simulink library "ESSLibrary"  (R2020a)
settings: Solver=VariableStepAuto  StartTime=0.0  StopTime=10.0  RelTol=1e-3
libraries: $bdroot x82, powerlib_meascontrol x10, simulink x7
(part 3 of 7)

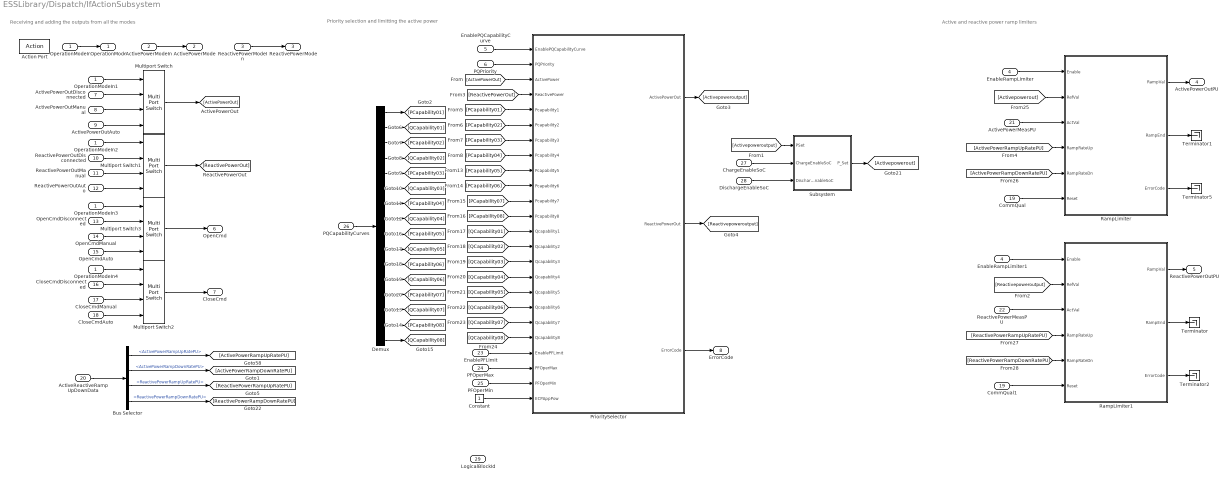
== system ESSLibrary/Dispatch/IfActionSubsystem ==
  note: Active and reactive power ramp limiters
  note: Priority selection and limitting the active power
  note: Receiving and adding the outputs from all the modes
  OperationModeIn : Inport  OutDataTypeStr=int8
  ActivePowerModeIn : Inport  Port=2
  ReactivePowerModeIn : Inport  Port=3
  EnableRampLimiter : Inport  Port=4
  EnablePQCapabilityCurve : Inport  Port=5
  PQPriority : Inport  Port=6
  ActivePowerOutDisconnected : Inport  Port=7
  ActivePowerOutManual : Inport  Port=8
  ActivePowerOutAuto : Inport  Port=9
  ReactivePowerOutDisconnected : Inport  Port=10
  ReactivePowerOutManual : Inport  Port=11
  ReactivePowerOutAuto : Inport  Port=12
  OpenCmdDisconnected : Inport  Port=13
  OpenCmdManual : Inport  Port=14
  OpenCmdAuto : Inport  Port=15
  CloseCmdDisconnected : Inport  Port=16
  CloseCmdManual : Inport  Port=17
  CloseCmdAuto : Inport  Port=18
  CommQual : Inport  Port=19
  ActiveReactiveRampUpDownData : Inport  Port=20  OutDataTypeStr=Bus: ActiveReactiveRampUpDownData
  ActivePowerMeasPU : Inport  Port=21
  ReactivePowerMeasPU : Inport  Port=22
  EnablePFLimit : Inport  Port=23
  PFOperMax : Inport  Port=24
  PFOperMin : Inport  Port=25
  PQCapabilityCurves : Inport  Port=26  OutDataTypeStr=double
  ChargeEnableSoC : Inport  Port=27
  DischargeEnableSoC : Inport  Port=28
  LogicalBlockId : Inport  Port=29
  Action Port : ActionPort
  Bus Selector : BusSelector  OutputSignals=ActivePowerRampUpRatePU,ActivePowerRampDownRatePU,ReactivePowerRampUpRatePU,ReactivePowerRampDownRatePU
  CommQual1 : InportShadow  Port=19
  Constant : Constant  OutDataTypeStr=double  SampleTime=-1
  Demux : Demux  Outputs=16
  EnableRampLimiter1 : InportShadow  Port=4
  Multiport Switch{,1..3} (4 alike) : MultiPortSwitch
  OperationModeIn{1..4} (4 alike) : InportShadow  OutDataTypeStr=int8
  PrioritySelector : Subsystem
  RampLimiter : MATLAB Function  TreatAsAtomicUnit=on
  RampLimiter1 : MATLAB Function  TreatAsAtomicUnit=on
  Subsystem : Subsystem
  Terminator{,1..2,5} (4 alike) : Terminator
  OperationMode : Outport
  ActivePowerMode : Outport  Port=2
  ReactivePowerMode : Outport  Port=3
  ActivePowerOutPU : Outport  Port=4
  ReactivePowerOutPU : Outport  Port=5
  OpenCmd : Outport  Port=6
  CloseCmd : Outport  Port=7
  ErrorCode : Outport  Port=8
  wires:
  Multiport Switch/1 -> [ActivePowerOut]
  Multiport Switch3/1 -> OpenCmd/1
  Multiport Switch1/1 -> [ReactivePowerOut]
  Multiport Switch2/1 -> CloseCmd/1
  OperationModeIn/1 -> OperationMode/1
  ActivePowerOutDisconnected/1 -> Multiport Switch/2
  ActivePowerOutManual/1 -> Multiport Switch/3
  ActivePowerOutAuto/1 -> Multiport Switch/4
  ReactivePowerOutAuto/1 -> Multiport Switch1/4
  ReactivePowerOutManual/1 -> Multiport Switch1/3
  ReactivePowerOutDisconnected/1 -> Multiport Switch1/2
  OpenCmdDisconnected/1 -> Multiport Switch3/2
  OpenCmdManual/1 -> Multiport Switch3/3
  OpenCmdAuto/1 -> Multiport Switch3/4
  CloseCmdAuto/1 -> Multiport Switch2/4
  CloseCmdManual/1 -> Multiport Switch2/3
  CloseCmdDisconnected/1 -> Multiport Switch2/2
  EnablePQCapabilityCurve/1 -> PrioritySelector/1(EnablePQCapabilityCurve)
  PQPriority/1 -> PrioritySelector/2(PQPriority)
  RampLimiter1/2(RampEnd) -> Terminator/1
  RampLimiter/3(ErrorCode) -> Terminator5/1
  RampLimiter/1(RampVal) -> ActivePowerOutPU/1
  EnableRampLimiter1/1 -> RampLimiter1/1(Enable)
  RampLimiter1/1(RampVal) -> ReactivePowerOutPU/1
  EnableRampLimiter/1 -> RampLimiter/1(Enable)
  PrioritySelector/1(ActivePowerOut) -> [Activepoweroutput]
  PrioritySelector/2(ReactivePowerOut) -> [Reactivepoweroutput]
  CommQual/1 -> RampLimiter/6(Reset)
  CommQual1/1 -> RampLimiter1/6(Reset)
  ActivePowerMeasPU/1 -> RampLimiter/3(ActVal)
  ReactivePowerMeasPU/1 -> RampLimiter1/3(ActVal)
  [ActivePowerOut] -> PrioritySelector/3(ActivePower)
  [ReactivePowerOut] -> PrioritySelector/4(ReactivePower)
  [ActivePowerRampUpRatePU] -> RampLimiter/4(RampRateUp)
  [ActivePowerRampDownRatePU] -> RampLimiter/5(RampRateDn)
  [ReactivePowerRampDownRatePU] -> RampLimiter1/5(RampRateDn)
  [ReactivePowerRampUpRatePU] -> RampLimiter1/4(RampRateUp)
  RampLimiter/2(RampEnd) -> Terminator1/1
  RampLimiter1/3(ErrorCode) -> Terminator2/1
  [Reactivepoweroutput] -> RampLimiter1/2(RefVal)
  EnablePFLimit/1 -> PrioritySelector/21(EnablePFLimit)
  PFOperMax/1 -> PrioritySelector/22(PFOperMax)
  PFOperMin/1 -> PrioritySelector/23(PFOperMin)
  PQCapabilityCurves/1 -> Demux/1
  Demux/1 -> [PCapability01]
  Demux/2 -> [QCapability01]
  Demux/3 -> [PCapability02]
  Demux/4 -> [QCapability02]
  Demux/5 -> [PCapability03]
  Demux/6 -> [QCapability03]
  Demux/7 -> [PCapability04]
  Demux/8 -> [QCapability04]
  Demux/9 -> [PCapability05]
  Demux/10 -> [QCapability05]
  Demux/11 -> [PCapability06]
  Demux/12 -> [QCapability06]
  Demux/13 -> [PCapability07]
  Demux/14 -> [QCapability07]
  Demux/15 -> [PCapability08]
  Demux/16 -> [QCapability08]
  [PCapability01] -> PrioritySelector/5(Pcapability1)
  [PCapability02] -> PrioritySelector/6(Pcapability2)
  [PCapability03] -> PrioritySelector/7(Pcapability3)
  [PCapability04] -> PrioritySelector/8(Pcapability4)
  [PCapability05] -> PrioritySelector/9(Pcapability5)
  [PCapability06] -> PrioritySelector/10(Pcapability6)
  [PCapability07] -> PrioritySelector/11(Pcapability7)
  [PCapability08] -> PrioritySelector/12(Pcapability8)
  [QCapability01] -> PrioritySelector/13(Qcapability1)
  [QCapability02] -> PrioritySelector/14(Qcapability2)
  [QCapability03] -> PrioritySelector/15(Qcapability3)
  [QCapability05] -> PrioritySelector/17(Qcapability5)
  [QCapability04] -> PrioritySelector/16(Qcapability4)
  [QCapability06] -> PrioritySelector/18(Qcapability6)
  [QCapability07] -> PrioritySelector/19(Qcapability7)
  [QCapability08] -> PrioritySelector/20(Qcapability8)
  [Activepoweroutput] -> Subsystem/1(PSet)
  ChargeEnableSoC/1 -> Subsystem/2(ChargeEnableSoC)
  DischargeEnableSoC/1 -> Subsystem/3(DischargeEnableSoC)
  [Activepowerout] -> RampLimiter/2(RefVal)
  PrioritySelector/3(ErrorCode) -> ErrorCode/1
  Subsystem/1(P_Set) -> [Activepowerout]
  ActivePowerModeIn/1 -> ActivePowerMode/1
  ReactivePowerModeIn/1 -> ReactivePowerMode/1
  Constant/1 -> PrioritySelector/24(ECPAppPow)
  OperationModeIn1/1 -> Multiport Switch/1
  OperationModeIn2/1 -> Multiport Switch1/1
  OperationModeIn3/1 -> Multiport Switch3/1
  OperationModeIn4/1 -> Multiport Switch2/1
  ActiveReactiveRampUpDownData/1 -> Bus Selector/1
  Bus Selector/1 -> [ActivePowerRampUpRatePU]  "<ActivePowerRampUpRatePU>"
  Bus Selector/2 -> [ActivePowerRampDownRatePU]  "<ActivePowerRampDownRatePU>"
  Bus Selector/3 -> [ReactivePowerRampUpRatePU]  "<ReactivePowerRampUpRatePU>"
  Bus Selector/4 -> [ReactivePowerRampDownRatePU]  "<ReactivePowerRampDownRatePU>"

== system ESSLibrary/Divider/ElseActionSubsystem ==
  Action Port : ActionPort
  Constant1 : Constant  Value=0  OutDataTypeStr=int64  SampleTime=-1
  Constant11 : Constant  Value=0  OutDataTypeStr=boolean  SampleTime=-1
  Constant2 : Constant  Value=0  OutDataTypeStr=double  SampleTime=-1
  Quality : Outport  OutDataTypeStr=boolean
  Out : Outport  Port=2  OutDataTypeStr=double
  ErrorCode : Outport  Port=3  OutDataTypeStr=int64
  wires:
  Constant2/1 -> Out/1
  Constant1/1 -> ErrorCode/1
  Constant11/1 -> Quality/1

== system ESSLibrary/Divider/IfActionSubsystem ==
  Numerator : Inport  OutDataTypeStr=double
  Denominator : Inport  Port=2  OutDataTypeStr=double
  Action Port : ActionPort
  Constant1 : Constant  OutDataTypeStr=int64  SampleTime=-1
  Constant11 : Constant  Value=0  SampleTime=-1
  Constant2 : Constant  Value=0  OutDataTypeStr=int64  SampleTime=-1
  Divide8 : Product  Inputs=*/
  NOT : Logic  Operator=NOT  IconShape=distinctive  AllPortsSameDT=off  OutDataTypeStr=boolean
  NOT1 : Logic  Operator=NOT  IconShape=distinctive  AllPortsSameDT=off  OutDataTypeStr=boolean
  Subsystem : Subsystem
  Switch1 : Switch  Criteria=u2 ~= 0
  Switch11 : Switch  Criteria=u2 ~= 0
  Quality : Outport  OutDataTypeStr=boolean
  Out : Outport  Port=2  OutDataTypeStr=double
  ErrorCode : Outport  Port=3  OutDataTypeStr=int64
  wires:
  [Quality2] -> NOT/1
  [Quality2] -> Quality/1
  Denominator/1 -> Subsystem/1(Denominator)
  [Divisor] -> Divide8/2
  NOT/1 -> Switch11/2
  Divide8/1 -> Switch11/1
  Constant1/1 -> Switch1/3
  Numerator/1 -> Divide8/1
  Constant2/1 -> Switch1/1
  Subsystem/2(Quality) -> [Quality2]
  NOT1/1 -> Switch1/2
  Constant11/1 -> Switch11/3
  [Quality2] -> NOT1/1
  Switch11/1 -> Out/1
  Subsystem/1(Divisor) -> [Divisor]
  Switch1/1 -> ErrorCode/1

== system ESSLibrary/DroopResponse_Points/If Action Subsystem ==
  ActVal : Inport
  Xdata : Inport  Port=2
  Ydata : Inport  Port=3
  Action Port : ActionPort
  MATLAB Function1 : MATLAB Function  TreatAsAtomicUnit=on
  Interpol : Outport
  ErrorCode : Outport  Port=2
  wires:
  MATLAB Function1/1(Interpol) -> Interpol/1
  ActVal/1 -> MATLAB Function1/1(ActVal)
  Xdata/1 -> MATLAB Function1/2(Xdata)
  Ydata/1 -> MATLAB Function1/3(Ydata)
  MATLAB Function1/2(ErrorCode) -> ErrorCode/1

== system ESSLibrary/DroopResponse_Points/If Action Subsystem2 ==
  Action Port : ActionPort
  Constant : Constant  Value=0  SampleTime=-1
  Out : Outport
  ErrorCode : Outport  Port=2
  wires:
  Constant/1 -> Out/1, ErrorCode/1

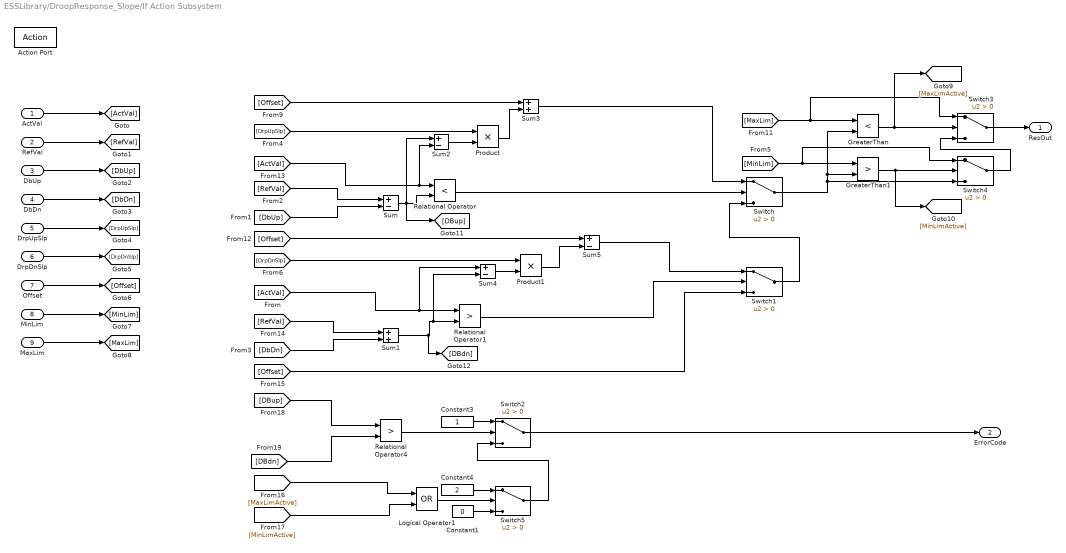
== system ESSLibrary/DroopResponse_Slope/If Action Subsystem ==
  ActVal : Inport
  RefVal : Inport  Port=2
  DbUp : Inport  Port=3
  DbDn : Inport  Port=4
  DrpUpSlp : Inport  Port=5
  DrpDnSlp : Inport  Port=6
  Offset : Inport  Port=7
  MinLim : Inport  Port=8
  MaxLim : Inport  Port=9
  Action Port : ActionPort
  Constant1 : Constant  Value=0
  Constant3 : Constant
  Constant4 : Constant  Value=2
  GreaterThan : RelationalOperator  Operator=<  OutDataTypeStr=boolean  RndMeth=Simplest
  GreaterThan1 : RelationalOperator  Operator=>  OutDataTypeStr=boolean  RndMeth=Simplest
  Logical Operator1 : Logic  Operator=OR  AllPortsSameDT=off  OutDataTypeStr=boolean
  Product : Product
  Product1 : Product
  Relational Operator : RelationalOperator  Operator=<  OutDataTypeStr=boolean  RndMeth=Simplest
  Relational Operator1 : RelationalOperator  Operator=>  OutDataTypeStr=boolean  RndMeth=Simplest
  Relational Operator4 : RelationalOperator  Operator=>  OutDataTypeStr=boolean  RndMeth=Simplest
  Sum{,2,4..5} (4 alike) : Sum  Inputs=+-
  Sum1 : Sum
  Sum3 : Sum
  Switch{,1..5} (6 alike) : Switch  Criteria=u2 > Threshold
  ResOut : Outport
  ErrorCode : Outport  Port=2
  wires:
  DrpUpSlp/1 -> [DrpUpSlp]
  DrpDnSlp/1 -> [DrpDnSlp]
  Offset/1 -> [Offset]
  RefVal/1 -> [RefVal]
  ActVal/1 -> [ActVal]
  DbUp/1 -> [DbUp]
  DbDn/1 -> [DbDn]
  Constant3/1 -> Switch2/1
  [DbUp] -> Sum/2
  [ActVal] -> Relational Operator1/1, Sum4/1
  Relational Operator1/1 -> Switch1/2
  [Offset] -> Switch1/3
  [Offset] -> Sum3/1
  Switch1/1 -> Switch/3
  Sum4/1 -> Product1/2
  Relational Operator/1 -> Switch/2
  [RefVal] -> Sum/1
  Sum3/1 -> Switch/1
  [RefVal] -> Sum1/1
  Switch5/1 -> Switch2/3
  Sum2/1 -> Product/2
  Sum5/1 -> Switch1/1
  Sum/1 -> [DBup], Relational Operator/2, Sum2/1
  [Offset] -> Sum5/1
  Product1/1 -> Sum5/2
  [DrpDnSlp] -> Product1/1
  Relational Operator4/1 -> Switch2/2
  [DbDn] -> Sum1/2
  Product/1 -> Sum3/2
  [ActVal] -> Relational Operator/1, Sum2/2
  Sum1/1 -> [DBdn], Relational Operator1/2, Sum4/2
  [DrpUpSlp] -> Product/1
  [DBup] -> Relational Operator4/1
  [DBdn] -> Relational Operator4/2
  Switch2/1 -> ErrorCode/1
  MinLim/1 -> [MinLim]
  MaxLim/1 -> [MaxLim]
  [MaxLim] -> Switch3/1, GreaterThan/1
  GreaterThan/1 -> [MaxLimActive], Switch3/2
  [MinLim] -> Switch4/1, GreaterThan1/1
  GreaterThan1/1 -> [MinLimActive], Switch4/2
  Switch4/1 -> Switch3/3
  Switch/1 -> GreaterThan/2, GreaterThan1/2, Switch4/3
  Switch3/1 -> ResOut/1
  Constant1/1 -> Switch5/3
  [MinLimActive] -> Logical Operator1/2
  Logical Operator1/1 -> Switch5/2
  Constant4/1 -> Switch5/1
  [MaxLimActive] -> Logical Operator1/1

== system ESSLibrary/DroopResponse_Slope/If Action Subsystem1 ==
  Action Port : ActionPort
  Constant : Constant  Value=0  SampleTime=-1
  ResOut : Outport
  ErrorCode : Outport  Port=2
  wires:
  Constant/1 -> ResOut/1, ErrorCode/1

== system ESSLibrary/DynamicVoltWattMode/MovAvgDeltaVoltCalc ==
  Enable : Inport
  Inp : Inport  Port=2
  FilterTime : Inport  Port=3
  TimeStep : Inport  Port=4
  ElseMovAvgFilter : Subsystem  TreatAsAtomicUnit=on
  If : If  IfExpression=u1 ~= 0
  IfMovAvgFilter : Subsystem  TreatAsAtomicUnit=on
  Inp1 : InportShadow  Port=2
  Switch : Switch  Criteria=u2 > Threshold
  Switch1 : Switch  Criteria=u2 > Threshold
  Out : Outport
  ErrorCode : Outport  Port=2
  wires:
  Enable/1 -> Switch1/2, Switch/2, If/1
  If/2 -> ElseMovAvgFilter/Action
  If/1 -> IfMovAvgFilter/Action
  Inp/1 -> IfMovAvgFilter/1(Inp)
  TimeStep/1 -> IfMovAvgFilter/3(TimeStep)
  FilterTime/1 -> IfMovAvgFilter/2(FilterTime)
  Inp1/1 -> ElseMovAvgFilter/1(Inp)
  ElseMovAvgFilter/1(Out) -> [ElseOut]
  ElseMovAvgFilter/2(ErrorCode) -> [ElseErrorCode]
  IfMovAvgFilter/1(Out) -> [IfOut]
  IfMovAvgFilter/2(ErrorCode) -> [IfErrorCode]
  Switch1/1 -> ErrorCode/1
  Switch/1 -> Out/1
  [ElseOut] -> Switch/3
  [IfOut] -> Switch/1
  [IfErrorCode] -> Switch1/1
  [ElseErrorCode] -> Switch1/3

== system ESSLibrary/FilterResponse/If Action Subsystem ==
  SignalIn : Inport
  LeadTmConst : Inport  Port=2
  LagTmConst : Inport  Port=3
  TimeStep : Inport  Port=4
  Action Port : ActionPort
  A*X(k)+B*u(k) : Sum  SaturateOnIntegerOverflow=on
  C*X(k)+D*u(k) : Sum  SaturateOnIntegerOverflow=on
  Constant1 : Constant
  Constant2 : Constant
  Constant3 : Constant
  Constant4 : Constant  Value=0
  Delay : Delay  DelayLength=1  InitialCondition=0
  Logical Operator1 : Logic  Operator=OR  IconShape=distinctive  AllPortsSameDT=off  OutDataTypeStr=boolean
  Product{1..4} (4 alike) : Product
  Subsystem1 : Subsystem
  Subsystem2 : Subsystem
  Sum : Sum  Inputs=+-  SaturateOnIntegerOverflow=on
  Sum2 : Sum  Inputs=+-  SaturateOnIntegerOverflow=on
  Switch38 : Switch  Criteria=u2 > Threshold  OutDataTypeStr=int64
  SignalOut : Outport  InitialOutput=0
  ErrorCode : Outport  Port=2  InitialOutput=0
  wires:
  Logical Operator1/1 -> Switch38/2
  Subsystem2/1(Quotient) -> Product4/2, Sum2/2
  Constant2/1 -> Sum2/1
  Sum2/1 -> Product1/1  "x(k)"
  Subsystem1/1(Quotient) -> Sum/2, Product2/2
  Product2/1 -> C*X(k)+D*u(k)/1
  Product1/1 -> A*X(k)+B*u(k)/2
  LagTmConst/1 -> Subsystem2/2(Denominator), Subsystem1/2(Denominator)
  Constant1/1 -> Sum/1
  TimeStep/1 -> Subsystem2/1(Numerator)
  Product4/1 -> A*X(k)+B*u(k)/1
  LeadTmConst/1 -> Subsystem1/1(Numerator)
  C*X(k)+D*u(k)/1 -> SignalOut/1  "y"
  Product3/1 -> C*X(k)+D*u(k)/2
  A*X(k)+B*u(k)/1 -> Delay/1  "y"
  Switch38/1 -> ErrorCode/1
  SignalIn/1 -> Product4/1, Product2/1
  Constant4/1 -> Switch38/3
  Sum/1 -> Product3/1  "y"
  Constant3/1 -> Switch38/1
  Subsystem1/2(Quality) -> [quality1]
  [quality1] -> Logical Operator1/1
  [quality2] -> Logical Operator1/2
  Subsystem2/2(Quality) -> [quality2]
  Delay/1 -> Product3/2, Product1/2

== system ESSLibrary/FilterResponse/If Action Subsystem1 ==
  SignalIn : Inport
  Action Port : ActionPort
  Constant : Constant  Value=0  SampleTime=-1
  SignalOut : Outport  InitialOutput=0
  ErrorCode : Outport  Port=2  InitialOutput=0
  wires:
  SignalIn/1 -> SignalOut/1
  Constant/1 -> ErrorCode/1

== system ESSLibrary/Manual/ElseActionSubsystem ==
  Action Port : ActionPort  ActionPortLabel=else
  Constant1 : Constant  Value=0  OutDataTypeStr=int64  SampleTime=-1
  Constant2 : Constant  Value=0  OutDataTypeStr=boolean  SampleTime=-1
  Constant6 : Constant  Value=0  OutDataTypeStr=double  SampleTime=-1
  ActivePowerOut : Outport  OutDataTypeStr=double
  ReactivePowerOut : Outport  Port=2  OutDataTypeStr=double
  OpenCmd : Outport  Port=3  OutDataTypeStr=boolean
  CloseCmd : Outport  Port=4  OutDataTypeStr=boolean
  ErrorCode : Outport  Port=5  OutDataTypeStr=int64
  wires:
  Constant1/1 -> ErrorCode/1
  Constant2/1 -> CloseCmd/1, OpenCmd/1
  Constant6/1 -> ReactivePowerOut/1, ActivePowerOut/1

== system ESSLibrary/Manual/IfActionSubsystem ==
  OpenCmdIn : Inport  OutDataTypeStr=boolean
  CloseCmdIn : Inport  Port=2  OutDataTypeStr=boolean
  FreqWithinLimits : Inport  Port=3  OutDataTypeStr=boolean
  VoltWithinLimits : Inport  Port=4  OutDataTypeStr=boolean
  ActivePowerSetPU : Inport  Port=5  OutDataTypeStr=double
  ReactivePowerSetPU : Inport  Port=6  OutDataTypeStr=double
  ZeroActivePowerFlow : Inport  Port=7  OutDataTypeStr=boolean
  ZeroReactivePowerFlow : Inport  Port=8  OutDataTypeStr=boolean
  CBStatus : Inport  Port=9  OutDataTypeStr=int8
  BreakerCmdTime : Inport  Port=10
  OpenTimeOut : Inport  Port=11
  CloseTimeOut : Inport  Port=12
  LogicalBlockID : Inport  Port=13  OutDataTypeStr=int64
  Action Port : ActionPort  ActionPortLabel=if(u1 ~= 0)
  Constant26 : Constant  Value=0  OutDataTypeStr=int64
  Constant27 : Constant  Value=0  OutDataTypeStr=int64
  Equal2 : RelationalOperator  Operator=>  OutDataTypeStr=boolean  RndMeth=Simplest
  Gain : Gain  Gain=1000000
  MATLAB Function : MATLAB Function  TreatAsAtomicUnit=on
  Sum2 : Sum  OutDataTypeStr=int64
  Switch1 : Switch  Criteria=u2 > Threshold
  ActivePowerOut : Outport
  ReactivePowerOut : Outport  Port=2
  OpenCmd : Outport  Port=3
  CloseCmd : Outport  Port=4
  ErrorCode : Outport  Port=5
  wires:
  MATLAB Function/3(OpenCmd) -> OpenCmd/1
  MATLAB Function/1(ActivePowerOut) -> ActivePowerOut/1
  MATLAB Function/2(ReactivePowerOut) -> ReactivePowerOut/1
  MATLAB Function/4(CloseCmd) -> CloseCmd/1
  Sum2/1 -> Switch1/1
  Constant26/1 -> Equal2/2
  MATLAB Function/5(ErrorCode) -> Equal2/1, Sum2/1
  Gain/1 -> Sum2/2
  LogicalBlockID/1 -> Gain/1
  Equal2/1 -> Switch1/2
  Constant27/1 -> Switch1/3
  Switch1/1 -> ErrorCode/1
  OpenCmdIn/1 -> MATLAB Function/1(OpenCmdIn)
  CloseCmdIn/1 -> MATLAB Function/2(CloseCmdIn)
  FreqWithinLimits/1 -> MATLAB Function/3(FreqWithinLimits)
  VoltWithinLimits/1 -> MATLAB Function/4(VoltWithinLimits)
  CBStatus/1 -> MATLAB Function/9(CBStatus)
  BreakerCmdTime/1 -> MATLAB Function/10(BreakerCmdTime)
  ActivePowerSetPU/1 -> MATLAB Function/5(ActivePowerSetPU)
  ZeroActivePowerFlow/1 -> MATLAB Function/7(ZeroActivePowerFlow)
  ReactivePowerSetPU/1 -> MATLAB Function/6(ReactivePoweSetPU)
  ZeroReactivePowerFlow/1 -> MATLAB Function/8(ZeroReactivePowerFlow)
  OpenTimeOut/1 -> MATLAB Function/11(OpenTimeOut)
  CloseTimeOut/1 -> MATLAB Function/12(CloseTimeOut)

== system ESSLibrary/MovAvgDeltaVoltCalc1/ElseMovAvgFilter ==
  Inp : Inport
  Action Port : ActionPort
  Constant : Constant  Value=0  OutDataTypeStr=int64  SampleTime=-1
  Out : Outport
  ErrorCode : Outport  Port=2
  wires:
  Inp/1 -> Out/1
  Constant/1 -> ErrorCode/1

== system ESSLibrary/MovAvgDeltaVoltCalc1/IfMovAvgFilter ==
  Inp : Inport
  FilterTime : Inport  Port=2
  TimeStep : Inport  Port=3
  Action Port : ActionPort
  Constant : Constant  Value=0
  Constant1 : Constant  Value=0
  DiscreteMovingAverage : MATLAB Function  TreatAsAtomicUnit=on
  Enabled Subsystem : Subsystem  TreatAsAtomicUnit=on
  Relational Operator : RelationalOperator  Operator=>  OutDataTypeStr=boolean  ZeroCross=off  RndMeth=Simplest
  Switch : Switch  Criteria=u2 > Threshold
  Out : Outport
  ErrorCode : Outport  Port=2
  wires:
  Inp/1 -> DiscreteMovingAverage/2(Inp)
  Constant/1 -> Relational Operator/2
  FilterTime/1 -> Enabled Subsystem/2(FilterTime)
  Switch/1 -> DiscreteMovingAverage/1(NoOfTS)
  Enabled Subsystem/1(NoOfTimeStep) -> Switch/1
  Relational Operator/1 -> Switch/2, Enabled Subsystem/Enable
  TimeStep/1 -> Enabled Subsystem/1(TimeStep), Relational Operator/1
  DiscreteMovingAverage/1(Out) -> Out/1
  Constant1/1 -> Switch/3

== system ESSLibrary/OperationModeSelector/ElseActionSubsystem ==
  Action Port : ActionPort
  Constant1 : Constant  Value=0  OutDataTypeStr=boolean  SampleTime=-1
  Constant2 : Constant  Value=0  OutDataTypeStr=boolean  SampleTime=-1
  Constant3 : Constant  Value=0  OutDataTypeStr=boolean  SampleTime=-1
  Constant4 : Constant  Value=0  OutDataTypeStr=int64  SampleTime=-1
  EnableDisconnected : Outport
  EnableManual : Outport  Port=2
  EnableAuto : Outport  Port=3
  ErrorCodeOut : Outport  Port=4  OutDataTypeStr=int64
  wires:
  Constant1/1 -> EnableManual/1
  Constant3/1 -> EnableAuto/1
  Constant2/1 -> EnableDisconnected/1
  Constant4/1 -> ErrorCodeOut/1

== system ESSLibrary/OperationModeSelector/IfAction Subsystem ==
  OperationMode : Inport  OutDataTypeStr=int8
  LogicalBlockID : Inport  Port=2  OutDataTypeStr=int64
  Action Port : ActionPort
  Comparator : Subsystem
  Constant1 : Constant  Value=4  OutDataTypeStr=int8
  Constant10 : Constant  Value=0  OutDataTypeStr=int64
  Constant11 : Constant  Value=0  OutDataTypeStr=int64
  Constant2 : Constant  Value=2  OutDataTypeStr=int32
  Constant3 : Constant  Value=0  OutDataTypeStr=int8
  Constant4 : Constant  Value=0  OutDataTypeStr=int8
  Constant5 : Constant  Value=0  OutDataTypeStr=int8
  Constant6 : Constant  OutDataTypeStr=boolean
  Constant8 : Constant  OutDataTypeStr=int8
  Constant9 : Constant  Value=2  OutDataTypeStr=int8
  Equal : RelationalOperator  Operator===  OutDataTypeStr=boolean  RndMeth=Simplest
  Equal1 : RelationalOperator  Operator===  OutDataTypeStr=boolean  RndMeth=Simplest
  Equal2 : RelationalOperator  Operator=>  OutDataTypeStr=boolean  RndMeth=Simplest
  Gain1 : Gain  Gain=1000000
  Logical Operator : Logic  AllPortsSameDT=off  OutDataTypeStr=boolean
  NOT : Logic  Operator=NOT  IconShape=distinctive  AllPortsSameDT=off  OutDataTypeStr=boolean
  NOT1 : Logic  Operator=NOT  IconShape=distinctive  AllPortsSameDT=off  OutDataTypeStr=boolean
  Sum1 : Sum  OutDataTypeStr=int64
  Switch4 : Switch  Criteria=u2 > Threshold
  Terminator : Terminator
  Terminator1 : Terminator
  VariableIdentifier : Constant  OutDataTypeStr=int64
  EnableDisconnected : Outport
  EnableManual : Outport  Port=2
  EnableAuto : Outport  Port=3
  ErrorCodeOut : Outport  Port=4  OutDataTypeStr=int64
  wires:
  OperationMode/1 -> Equal1/1, Comparator/2("Input "), Equal/1
  Equal/1 -> NOT/1, EnableDisconnected/1
  Equal1/1 -> NOT1/1, EnableManual/1
  Logical Operator/1 -> EnableAuto/1
  Constant8/1 -> Equal/2
  Constant9/1 -> Equal1/2
  NOT/1 -> Logical Operator/1
  NOT1/1 -> Logical Operator/2
  Constant6/1 -> Comparator/1(Enable/Disable)
  Constant1/1 -> Comparator/3(UpperTrhd)
  Constant4/1 -> Comparator/4(LowerTrhd)
  Constant2/1 -> Comparator/5(HystSelection)
  Constant3/1 -> Comparator/6(AbsHyst)
  Constant5/1 -> Comparator/7(RelHyst)
  VariableIdentifier/1 -> Comparator/8(VariableIdentifier)
  Constant11/1 -> Switch4/3
  Constant10/1 -> Equal2/2
  Switch4/1 -> ErrorCodeOut/1
  Comparator/1(ErrorCode) -> Equal2/1, Sum1/1
  Equal2/1 -> Switch4/2
  Sum1/1 -> Switch4/1
  LogicalBlockID/1 -> Gain1/1
  Gain1/1 -> Sum1/2
  Comparator/2(MaxLimitCrossed) -> Terminator/1
  Comparator/3(MinLimitCrossed) -> Terminator1/1

== system ESSLibrary/PFReference_P/If Action Subsystem ==
  PFLimit : Inport
  PValPFLimit : Inport  Port=2
  PValPF1 : Inport  Port=3
  PSet : Inport  Port=4
  Action Port : ActionPort
  Basic alarm ver1.0 : Subsystem
  Constant1 : Constant  Value=16  SampleTime=-1
  Constant19 : Constant  Value=32  SampleTime=-1
  Constant2 : Constant  OutDataTypeStr=int32
  Constant20 : Constant  Value=0  SampleTime=-1
  Constant3 : Constant  OutDataTypeStr=boolean
  Constant4 : Constant  OutDataTypeStr=boolean
  Constant5 : Constant  Value=0  SampleTime=-1
  Constant6 : Constant  OutDataTypeStr=boolean
  Constant7 : Constant  Value=0  OutDataTypeStr=int32
  Constant8 : Constant  Value=0  OutDataTypeStr=int32
  Divide1 : Product  Inputs=**
  Divide2 : Product  Inputs=**
  GreaterThan : RelationalOperator  Operator=>  OutDataTypeStr=boolean  RndMeth=Simplest
  Safe Divider : Subsystem  Description=|
      | This function divides input values accounting for a predefined dead band for denominator to avoid occurrence of divide by zero condition. 
      | If the input for denominator is inside the dead band then the function returns predefined output with quality bit as one. 
      | If input value for denominator is in the normal range, the function returns the calculated quotient with quality bit as zero.
  Sum1 : Sum  Inputs=|+-
  Sum2 : Sum  Inputs=|+-
  Sum5 : Sum
  Sum6 : Sum  Inputs=+-+
  Switch : Switch  Criteria=u2 ~= 0
  Switch1 : Switch  Criteria=u2 > Threshold
  Switch6 : Switch  Criteria=u2 > Threshold
  Switch8 : Switch  Criteria=u2 ~= 0
  Terminator1 : Terminator
  Terminator2 : Terminator
  Terminator4 : Terminator
  UnityPF : Constant
  PFSet : Outport
  ErrorCode : Outport  Port=2
  wires:
  UnityPF/1 -> Sum1/2
  PValPFLimit/1 -> Sum2/1, [PNomPFLimPU]
  PValPF1/1 -> Divide2/2, Sum2/2, [PNomPF1PU]
  Constant3/1 -> Safe Divider/1(Enable)
  Sum1/1 -> Safe Divider/2(Numerator)
  Sum2/1 -> Safe Divider/3(Denominator)
  Safe Divider/3(ErrorCode) -> Terminator2/1
  Safe Divider/2(Quality) -> Terminator1/1
  Safe Divider/1(Quotient) -> Divide2/1, Divide1/2
  Switch/1 -> Divide1/1
  Constant6/1 -> Basic alarm ver1.0/1(Enable/disable)
  PSet/1 -> Basic alarm ver1.0/2("Input "), [Pset]
  Constant2/1 -> Basic alarm ver1.0/5(HystSelection)
  Constant7/1 -> Basic alarm ver1.0/6(AbsHyst)
  Constant8/1 -> Basic alarm ver1.0/7(RelHyst)
  Basic alarm ver1.0/1("Output ") -> Switch1/2, Switch/2, [PSetRange]
  [Pset] -> Switch/3
  Switch1/1 -> Switch/1
  Basic alarm ver1.0/2(ErrorCode) -> Terminator4/1
  [PNomPF1PU] -> GreaterThan/1
  [PNomPFLimPU] -> GreaterThan/2
  Sum5/1 -> ErrorCode/1
  PFLimit/1 -> Sum1/1, [PFLimt]
  GreaterThan/1 -> Switch6/2
  Constant1/1 -> Switch6/1
  Constant5/1 -> Switch6/3
  Switch6/1 -> Sum5/1
  Divide1/1 -> Sum6/1
  Divide2/1 -> Sum6/2
  Constant4/1 -> Sum6/3
  Sum6/1 -> PFSet/1
  [PSetRange] -> Switch8/2
  Constant19/1 -> Switch8/1
  Switch8/1 -> Sum5/2
  Constant20/1 -> Switch8/3
  [PNomPF1PU] -> Basic alarm ver1.0/3(UpperTrhd)
  [PNomPFLimPU] -> Basic alarm ver1.0/4(LowerTrhd)
  [PNomPF1PU] -> Switch1/1
  [PNomPFLimPU] -> Switch1/3

== system ESSLibrary/PFReference_P/If Action Subsystem1 ==
  Action Port : ActionPort
  Constant : Constant  Value=0  SampleTime=-1
  ElsePFSet : Outport
  ErrorCode : Outport  Port=2
  wires:
  Constant/1 -> ErrorCode/1, ElsePFSet/1

== system ESSLibrary/PIController/If Action Subsystem ==
  ErrSig : Inport
  Kp : Inport  Port=2
  Ki : Inport  Port=3
  TimeStep : Inport  Port=4
  HighLimit : Inport  Port=5
  LowLimit : Inport  Port=6
  Action Port : ActionPort  InitializeStates=reset
  " " : RelationalOperator  Operator=<=  OutDataTypeStr=boolean  RndMeth=Simplest
  Add : Sum
  Add1 : Sum
  Constant : Constant  Value=0.0  OutDataTypeStr=double
  Constant7 : Constant  OutDataTypeStr=int32  SampleTime=-1
  Constant8 : Constant  Value=2  OutDataTypeStr=int32  SampleTime=-1
  Delay : Delay  DelayLength=1  InitialCondition=0
  Delay1 : Delay  DelayLength=1  InitialConditionSource=Input port  InitialCondition=0
      settings: InputPortMap=u0,p4
  Less Than1 : RelationalOperator  OutDataTypeStr=boolean  RndMeth=Simplest
  Logical Operator : Logic  Operator=OR  AllPortsSameDT=off  OutDataTypeStr=boolean
  Product : Product
  Product1 : Product  Inputs=3
  Switch : Switch  Criteria=u2 > Threshold
  Switch1 : Switch  Criteria=u2 > Threshold
  Switch2 : Switch  Criteria=u2 > Threshold
  CntrSig : Outport
  ErrorCode : Outport  Port=2
  wires:
  TimeStep/1 -> Product1/3
  ErrSig/1 -> Delay/1, Product/1
  Ki/1 -> Product1/2
  Add1/1 -> Switch1/3, Less Than1/2, " "/2
  Product1/1 -> Add/1
  Add/1 -> Add1/2
  Delay1/1 -> Add/2
  Product/1 -> Add1/1
  HighLimit/1 -> Switch/1, " "/1
  LowLimit/1 -> Less Than1/1, Switch1/1
  Delay/1 -> Product1/1
  Kp/1 -> Product/2
  Constant/1 -> Delay1/2
  " "/1 -> [MaxCheck], Switch/2
  Less Than1/1 -> [MinCheck], Switch1/2
  Switch1/1 -> Switch/3
  Switch/1 -> Delay1/1, CntrSig/1
  Logical Operator/1 -> Switch2/2
  [MinCheck] -> Logical Operator/2
  Switch2/1 -> ErrorCode/1
  [MaxCheck] -> Logical Operator/1
  Constant8/1 -> Switch2/3
  Constant7/1 -> Switch2/1

== system ESSLibrary/PIController/If Action Subsystem1 ==
  Action Port : ActionPort  InitializeStates=reset
  Constant : Constant  Value=0  SampleTime=-1
  Out : Outport  InitialOutput=0
  ErrorCode : Outport  Port=2
  wires:
  Constant/1 -> ErrorCode/1, Out/1

== system ESSLibrary/PostProcessing/ElseActionSubsystem ==
  Action Port : ActionPort
  Constant1 : Constant  Value=0  OutDataTypeStr=double  SampleTime=-1
  ActivePowerOut : Outport
  ReactivePowerOut : Outport  Port=2
  wires:
  Constant1/1 -> ReactivePowerOut/1, ActivePowerOut/1

== system ESSLibrary/PostProcessing/If Action Subsystem ==
  ECPAppPow : Inport
  ActivePowerPU : Inport  Port=2
  ReactivePowerPU : Inport  Port=3
  Action Port : ActionPort
  Divide : Product  Inputs=**
  Divide1 : Product  Inputs=**
  ActivePowerOut : Outport
  ReactivePowerOut : Outport  Port=2
  wires:
  ActivePowerPU/1 -> Divide/2
  ReactivePowerPU/1 -> Divide1/2
  ECPAppPow/1 -> Divide1/1, Divide/1
  Divide/1 -> ActivePowerOut/1
  Divide1/1 -> ReactivePowerOut/1

== system ESSLibrary/PreProcessing/ElseActionSubsystem ==
  Action Port : ActionPort
  Constant1 : Constant  Value=[0.0 0.0 0.0 0.0]  OutDataTypeStr=Bus: Active_ReactiveRampUp_DownData  SampleTime=-1
  Constant10 : Constant  Value=[0.0 0.0 0.0 0.0 0.0 0.0 0.0 0.0 0.0 0.0]  OutDataTypeStr=Bus: VoltWattOperatingParametersPU  SampleTime=-1
  Constant11 : Constant  Value=[0.0 0.0 0.0 0.0 0.0 0.0 0.0 0.0 0.0 0.0]  OutDataTypeStr=Bus: FreqWattOperatingParametersPU  SampleTime=-1
  Constant12 : Constant  Value=[0.0 0.0 0.0 0.0 0.0]  OutDataTypeStr=Bus: DynamicVoltWattOperatingParameters  SampleTime=-1
  Constant13 : Constant  Value=[0.0 0.0 0.0 0.0 0.0 0.0 0.0]  OutDataTypeStr=Bus: VoltVarOperatingParametersPU  SampleTime=-1
  Constant14 : Constant  Value=[0.0 0.0 0.0 0.0 0.0 0.0 0.0]  OutDataTypeStr=Bus: WattVarOperatingParametersPU  SampleTime=-1
  Constant15 : Constant  Value=0  OutDataTypeStr=int16
  Constant2 : Constant  Value=0  OutDataTypeStr=double
  Constant3 : Constant  Value=0  OutDataTypeStr=boolean
  Constant4 : Constant  Value=[0.0 0.0 0.0 0.0 0.0 0.0 0.0 0.0 0.0 0.0 0.0 0.0 0.0 0.0 0.0 0.0]  OutDataTypeStr=double  SampleTime=-1
  Constant5 : Constant  Value=0  OutDataTypeStr=boolean
  Constant6 : Constant  Value=[0.0 0.0]  OutDataTypeStr=Bus: ActivePowerLimitOperatingParametersPU  SampleTime=-1
  Constant7 : Constant  Value=[0.0 0.0 0.0 0.0 0.0]  OutDataTypeStr=Bus: CrdChargeDischargeOperatingParametersPU  SampleTime=-1
  Constant8 : Constant  Value=[0.0 0.0 0.0]  OutDataTypeStr=Bus: ActivePowerResponseOperatingParametersPU  SampleTime=-1
  Constant9 : Constant  Value=[0.0 0.0 0.0 0.0 0.0]  OutDataTypeStr=Bus: ActivePowerSmoothingOperatingParametersPU  SampleTime=-1
  ActivePowerSetPU : Outport
  "ReactivePowerSetPU " : Outport  Port=2
  ActivePowerMeasPU : Outport  Port=3
  ReactivePowerMeasPU : Outport  Port=4
  ActivePowerMeasCtrlPointPU : Outport  Port=5
  ReactivePowerMeasCtrlPointPU : Outport  Port=6
  FreqMeasPU : Outport  Port=7
  VoltMeasPU : Outport  Port=8
  MaxDischargingPowerPU : Outport  Port=9
  MaxChargingPowerPU : Outport  Port=10
  FreqWithinLimits : Outport  Port=11
  VoltWithinLimits : Outport  Port=12
  Active_ReactiveRampUp_DownData : Outport  Port=13  OutDataTypeStr=Bus: Active_ReactiveRampUp_DownData
  FreqWattOperatingParametersPU : Outport  Port=14  OutDataTypeStr=Bus: FreqWattOperatingParametersPU
  DynamicVoltWattOperatingParametersPU : Outport  Port=15  OutDataTypeStr=Bus: DynamicVoltWattOperatingParameters
  VoltWattOperatingParametersPU : Outport  Port=16  OutDataTypeStr=Bus: VoltWattOperatingParametersPU
  ActivePowerSmoothingParametersPU : Outport  Port=17  OutDataTypeStr=Bus: ActivePowerSmoothingOperatingParametersPU
  ActivePowerResponseOperatingParametersPU : Outport  Port=18  OutDataTypeStr=Bus: ActivePowerResponseOperatingParametersPU
  CrdChargeDischargeOperatingParametersPU : Outport  Port=19  OutDataTypeStr=Bus: CrdChargeDischargeOperatingParametersPU
  ActivePowerLimitOperatingParametersPU : Outport  Port=20  OutDataTypeStr=Bus: ActivePowerLimitOperatingParametersPU
  WattVAROperatingParametersPU : Outport  Port=21  OutDataTypeStr=Bus: WattVarOperatingParametersPU
  VoltVAROperatingParametersPU : Outport  Port=22  OutDataTypeStr=Bus: VoltVarOperatingParametersPU
  ZeroActivePowerFlow : Outport  Port=23
  ZeroReactivePowerFlow : Outport  Port=24
  PQCapabiltyCurvePU : Outport  Port=25  OutDataTypeStr=double
  ErrorCode : Outport  Port=26
  BreakerCmdTimeSteps : Outport  Port=27
  OpenTimeOutTimeSteps : Outport  Port=28
  CloseTimeOutTimeSteps : Outport  Port=29
  wires:
  Constant3/1 -> ErrorCode/1
  Constant2/1 -> ActivePowerSetPU/1, "ReactivePowerSetPU "/1, ActivePowerMeasPU/1, ReactivePowerMeasPU/1, ActivePowerMeasCtrlPointPU/1, ReactivePowerMeasCtrlPointPU/1, FreqMeasPU/1, VoltMeasPU/1, MaxDischargingPowerPU/1, MaxChargingPowerPU/1
  Constant1/1 -> Active_ReactiveRampUp_DownData/1
  Constant4/1 -> PQCapabiltyCurvePU/1
  Constant5/1 -> VoltWithinLimits/1, FreqWithinLimits/1, ZeroReactivePowerFlow/1, ZeroActivePowerFlow/1
  Constant6/1 -> ActivePowerLimitOperatingParametersPU/1
  Constant7/1 -> CrdChargeDischargeOperatingParametersPU/1
  Constant8/1 -> ActivePowerResponseOperatingParametersPU/1
  Constant9/1 -> ActivePowerSmoothingParametersPU/1
  Constant10/1 -> VoltWattOperatingParametersPU/1
  Constant11/1 -> FreqWattOperatingParametersPU/1
  Constant12/1 -> DynamicVoltWattOperatingParametersPU/1
  Constant13/1 -> VoltVAROperatingParametersPU/1
  Constant14/1 -> WattVAROperatingParametersPU/1
  Constant15/1 -> CloseTimeOutTimeSteps/1, OpenTimeOutTimeSteps/1, BreakerCmdTimeSteps/1
